simulink model "pathPlanningSimulinkModel"  (R2020a)
settings: Solver=VariableStepAuto  StartTime=0.0  StopTime=inf  RelTol=1e-3
PostLoadFcn:
  | set_param(gcs, 'ForceConsistencyChecking', 'off');
InitFcn:
  | set_param('pathPlanningSimulinkModel', 'ForceConsistencyChecking', 'off')
model workspace (MAT data in the model file):
  Sig = Simulink.Signal
  Sig.DataType = 'auto'
  Sig.Dimensions = -1
  Sig.DimensionsMode = 'auto'
  Sig.Complexity = 'auto'
  Sig.SampleTime = -1
  Sig.SamplingMode = 'auto'
values from neighbouring files (symbols this model uses):
  goalLoc = [20 20]    [start.m]
  startLoc = [5 5]    [start.m]
undefined symbols (not defined in the file or in its folder): Angular, Linear, simpleMap
libraries: robotlib x3, simulink x1, robotalgslib x1
settings Model: OrderedModelArguments=off  Creator=The MathWorks, Inc.  LastModifiedBy=johni
settings DebuggingCC: SymbolicDimsDataTypeCodeGenerationDiagnostic=none

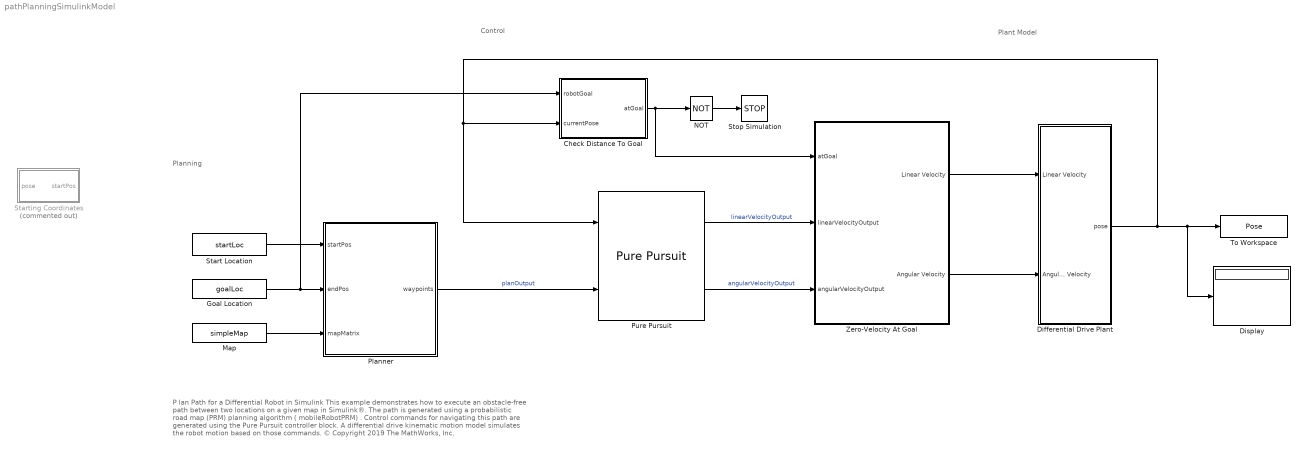
== system pathPlanningSimulinkModel ==
  note: Plant Model
  note: Control
  note: Planning
  note: P lan Path for a Differential Robot in Simulink
      | This example demonstrates how to execute an obstacle-free path between two locations on a given map in Simulink®. The path is generated using a probabilistic road map (PRM) planning algorithm ( mobileRobotPRM) . Control commands for navigating this path are generated using the Pure Pursuit controller block. A differential drive kinematic motion model simulates the robot motion based on those commands.
      |
      | © Copyright 2019 The MathWorks, Inc.
  Check Distance To Goal : Subsystem
  Differential Drive Plant : Subsystem
  Display : Display
  Goal Location : Constant  Value=goalLoc
  Map : Constant  Value=simpleMap
  NOT : Logic  Operator=NOT  IconShape=distinctive  AllPortsSameDT=off  OutDataTypeStr=boolean
  Planner : MATLAB Function  TreatAsAtomicUnit=on
  Pure Pursuit : robotalgslib/Pure Pursuit  DesiredLinearVelocity=2  MaxAngularVelocity=1.0  LookaheadDistance=0.5  TargetDirPort=off  SimulateUsing=Code generation
  Start Location : Constant  Value=startLoc
  Starting Coordinates : Subsystem  Commented=on
  Stop Simulation : Stop
  To Workspace : ToWorkspace  VariableName=Pose  SampleTime=-1
  Zero-Velocity At Goal : Subsystem
  wires:
  Check Distance To Goal/1(atGoal) -> Zero-Velocity At Goal/1(atGoal), NOT/1
  Pure Pursuit/1 -> Zero-Velocity At Goal/2(linearVelocityOutput)  "linearVelocityOutput"
  Planner/1(waypoints) -> Pure Pursuit/2  "planOutput"
  Pure Pursuit/2 -> Zero-Velocity At Goal/3(angularVelocityOutput)  "angularVelocityOutput"
  Goal Location/1 -> Check Distance To Goal/1(robotGoal), Planner/2(endPos)
  Map/1 -> Planner/3(mapMatrix)
  Differential Drive Plant/1(pose) -> To Workspace/1, Display/1, Pure Pursuit/1, Check Distance To Goal/2(currentPose)
  NOT/1 -> Stop Simulation/1
  Zero-Velocity At Goal/1(Linear Velocity) -> Differential Drive Plant/1(Linear Velocity)
  Zero-Velocity At Goal/2(Angular Velocity) -> Differential Drive Plant/2(Angular Velocity)
  Start Location/1 -> Planner/1(startPos)

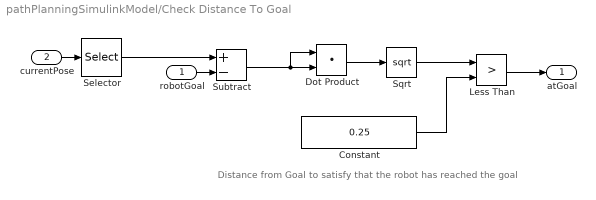
== system pathPlanningSimulinkModel/Check Distance To Goal ==
  note: Distance from Goal to satisfy that the robot has reached the goal
  robotGoal : Inport
  currentPose : Inport  Port=2
  Constant : Constant  Value=0.25
  Dot Product : DotProduct  InputSameDT=on  OutDataTypeStr=Inherit: Inherit via internal rule
  Less Than : RelationalOperator  Operator=>  OutDataTypeStr=boolean  RndMeth=Simplest
  Selector : Selector  InputPortWidth=3  IndexOptions=Index vector (dialog)  Indices=[1 2]  OutputSizes=1
  Sqrt : Sqrt  SaturateOnIntegerOverflow=on
  Subtract : Sum  Inputs=+-
  atGoal : Outport
  wires:
  robotGoal/1 -> Subtract/2
  Dot Product/1 -> Sqrt/1
  Constant/1 -> Less Than/2
  currentPose/1 -> Selector/1
  Less Than/1 -> atGoal/1
  Sqrt/1 -> Less Than/1
  Subtract/1 -> Dot Product/1, Dot Product/2
  Selector/1 -> Subtract/1

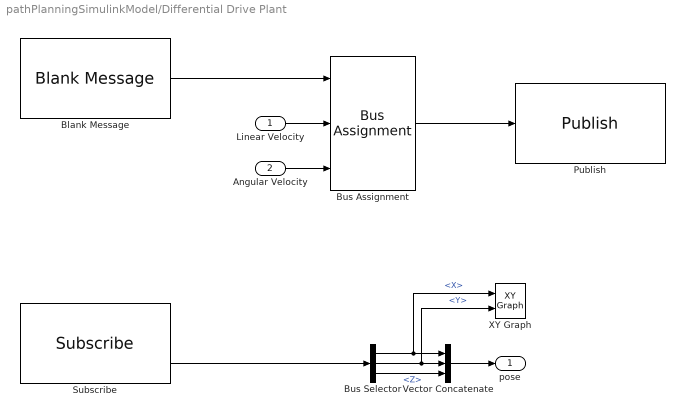
== system pathPlanningSimulinkModel/Differential Drive Plant ==
  Linear Velocity : Inport
  Angular Velocity : Inport  Port=2
  Blank Message : robotlib/Blank Message  messageClass=Message  entityType=geometry_msgs/Twist  messageType=geometry_msgs/Twist  SampleTime=0.01
  Bus Assignment : BusAssignment  AssignedSignals=Linear.X,Angular.Z
  Bus Selector : BusSelector  OutputSignals=Pose.Pose.Position.X,Pose.Pose.Position.Y,Pose.Pose.Orientation.Z
  Publish : robotlib/Publish  topicSource=Select from ROS network  topic=/mobile_base_controller/cmd_vel  messageType=geometry_msgs/Twist  messageQueueLength=1
  Subscribe : robotlib/Subscribe  topicSource=Select from ROS network  topic=/mobile_base_controller/odom  messageType=nav_msgs/Odometry  sampleTime=-1  messageQueueLength=1
  Vector Concatenate : Concatenate  NumInputs=3
  XY Graph : simulink/Sinks/XY Graph  xmin=-20  xmax=20  ymin=-20  ymax=20  st=-1
  pose : Outport
  wires:
  Blank Message/1 -> Bus Assignment/1
  Bus Assignment/1 -> Publish/1
  Linear Velocity/1 -> Bus Assignment/2
  Angular Velocity/1 -> Bus Assignment/3
  Subscribe/2 -> Bus Selector/1
  Bus Selector/1 -> XY Graph/1, Vector Concatenate/1  "<X>"
  Bus Selector/2 -> XY Graph/2, Vector Concatenate/2  "<Y>"
  Bus Selector/3 -> Vector Concatenate/3  "<Z>"
  Vector Concatenate/1 -> pose/1

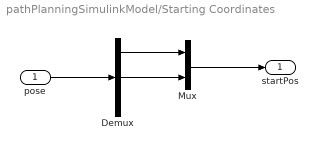
== system pathPlanningSimulinkModel/Starting Coordinates ==
  pose : Inport
  Demux : Demux  Outputs=3
  Mux : Mux  Inputs=2
  startPos : Outport
  wires:
  pose/1 -> Demux/1
  Demux/2 -> Mux/2
  Demux/1 -> Mux/1
  Mux/1 -> startPos/1

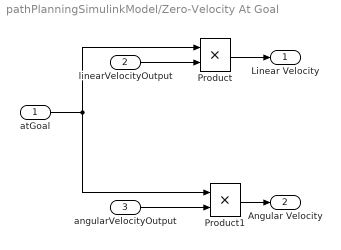
== system pathPlanningSimulinkModel/Zero-Velocity At Goal ==
  atGoal : Inport
  linearVelocityOutput : Inport  Port=2
  angularVelocityOutput : Inport  Port=3
  Product : Product
  Product1 : Product
  Linear Velocity : Outport  OutDataTypeStr=double
  Angular Velocity : Outport  Port=2  OutDataTypeStr=double
  wires:
  atGoal/1 -> Product1/1, Product/1
  angularVelocityOutput/1 -> Product1/2
  linearVelocityOutput/1 -> Product/2
  Product/1 -> Linear Velocity/1
  Product1/1 -> Angular Velocity/1

== matlab function pathPlanningSimulinkModel/Planner ==
  settings: updateMethod=DISCRETE
  data: startPos input size=[1 2]; endPos input size=[1 2]; waypoints output size=[100 2]; mapMatrix input
function waypoints = planning(startPos, endPos, mapMatrix)

persistent waypointsInternal
persistent prevStartPos
persistent prevEndPos

% Set constant parameters
maxNumNodes = 100;

% Initialize persistent variables that are used downstream
if isempty(prevStartPos)
    prevStartPos = startPos;
end

if isempty(prevEndPos)
    prevEndPos = endPos;
end

isNewPath = (~isequal(prevStartPos, startPos) || ~isequal(prevEndPos, endPos));

if isempty(waypointsInternal) || isNewPath
    % Two conditions in which waypoints must be set: they are not yet
    % initialized, or they are initialized, but the current start and end
    % do not match those used to generate the previous set of waypoints
    [waypointsInternal] = planPath(mapMatrix, maxNumNodes, startPos, endPos);
end

% Update the outputs
waypoints = waypointsInternal;

% Update the persistent variables that indicate previous state
prevStartPos = startPos;
prevEndPos = endPos;

%% Helper Function

function wayPoints = planPath(mapMatrix, maxNodes, startPos, endPos)
    
    % Create a probabilistic roadmap
    map = binaryOccupancyMap(mapMatrix);
    prm = mobileRobotPRM(map, maxNodes);
    
    % Find a path between two points
    xy = findpath(prm, startPos, endPos);
    wayPoints = repmat(endPos, maxNodes, 1);
    
    % Number of nodes that are actually used
    numNodes = length(xy);
    wayPoints(1:numNodes,:) = xy;    

end

end
